simulink model "RealSim_UA_01"  (Simulink 10.0)
settings: Solver=ode1  StartTime=0.0  StopTime=Inf  FixedStep=0.001  RelTol=1e-3  EnableMultiTasking=on
PreLoadFcn:
  | if ~length(which('cmcmd')), cmenv; end
PostLoadFcn:
  | if any(exist('dsrtsu_mdlpostloadfcn', 'file') ~= 0), dsrtsu_mdlpostloadfcn('Execute', bdroot); end
InitFcn:
  | , if any(exist('dsmpb_private', 'file') ~= 0), dsmpb_private('dsmpb_mdlclblib', 'Init', bdroot); end,
undefined symbols (not defined in the file or in its folder): SUMONoDyn_SpeedFromSumo_mps, SUMONoDyn_Time_s
libraries: dsmpblib x7, simulink x4
PreSaveFcn:
  | , if any(exist('dsmpb_private', 'file') ~= 0), dsmpb_private('dsmpb_mdlclblib', 'PreSave', bdroot); end,
CloseFcn:
  | , if any(exist('dsmpb_private', 'file') ~= 0), dsmpb_private('dsmpb_mdlclblib', 'Close', bdroot); end,
settings Model: RTICANMMDATA=struct('GeneralSetupData',struct('modelroot','C:\ORNL\Code\cm10_realsim_UA_proj\src_cm4sl','generalsettings',struct('filesettings',struct('destfolder',struct('Name','RTICANMM_FILES','Check',1),'buildfolder',struct('Name','.','Check',1),'AbsDestfolder',struct('Name','C:\ORNL\Code\cm10_realsim_UA_proj\src_cm4sl\RTICANMM_FILES'),'AbsBuildfolder',struct('Name','C:\ORNL\Code\cm10_realsim_UA_proj\src_cm4sl'))),'options',struct('addpaths',1,'rmpaths',1,'addtrcexclusion',true,'cannavigator',struct('checkmonitoring',0),'show_usrtrc',0,'use_usrtrc',0),'advanced',struct('options',ones(1,100)),'MPSetup',{{}},'RTI',struct('Type','DSRT','Ver','4.2p1','Date','11-Feb-2020'),'modelname','RealSim_UA_01','block','RealSim_UA_01'))  DSRTSU_INTERNAL_RTIFPGA=150  DSMPB_ID_DATA={'3989',struct('BlockId','8a5b4871-e5f6-4132-a2a0-cfdc08ce5a62','SignalIds',{{'f768e98f-af3a-45f5-b8cc-d45140bad16b'}}),'3990',struct('BlockId','8935c71e-55a2-4122-9d8c-9a702d74f083','SignalIds',{{'7beae7fa-5028-4068-8a6f-9b12f3c7f2cd'}}),'3991',struct('BlockId','27d609ef-4027-4865-90b1-f647bdc0d63f','SignalIds',{{'f3b1d4b1-f31f-4d63-9d34-50172078722b','1a0ed1f8-b245-431e-8944-1442373f7090'}}),'3992',struct('BlockId','4d452e4e-1d5d-452d-b859-8d5b2ee4f974','SignalIds',{{'341be20d-510e-43ce-bf93-db3744e3af54','92dd9c2e-376e-43cb-936f-8d32abdccb4f','85825f80-a60d-4715-affe-6d21e145415d','eb0678fd-503c-45b4-9ef8-2c00783b7cf9'}}),'3994',struct('BlockId','13483ad7-c9a4-44e5-950b-a5cc0e7666e2','SignalIds',{{'3f16ee9e-b6cb-44ff-9801-e0155d01597e','6edf7b02-435e-4d6a-b940-049f7bb34941'}}),'3995',struct('BlockId','400b85df-e7bd-4fe3-9c0f-59686a376489','SignalIds',{{'36519bb0-7faf-46a8-b3e5-661b8781a7f8'}}),'4054',struct('BlockId','353e6fb8-1188-4f2a-93b8-42c0e6c342a3','SignalIds',{{'0c3ec644-6183-447e-85a0-984a42e1fc9b'}})}  Creator=fh  LastModifiedBy=Paul_User  ExtModeAutoUpdateStatusClock=off
settings DataIOCC: LimitDataPoints=on  SignalLoggingName=sigsOut
settings OptimizationCC: BlockReduction=off  BooleanDataType=off  ConditionallyExecuteInputs=off  OptimizeBlockIOStorage=off  BufferReuse=off  GlobalBufferReuse=off  ExpressionFolding=off  ExpressionDepthLimit=2147483647  LocalBlockOutputs=off  InitFltsAndDblsToZero=on  LifeSpan=auto  OptimizeDataStoreBuffers=off  BusAssignmentInplaceUpdate=off
settings DebuggingCC: SaveWithParameterizedLinksMsg=none  SignalResolutionControl=TryResolveAllWithWarning  MultiTaskDSMMsg=warning  MultiTaskCondExecSysMsg=none  TasksWithSamePriorityMsg=none  FcnCallInpInsideContextMsg=warning  StateNameClashWarn=warning  SFExecutionAtInitializationDiag=warning
settings HardwareCC: ProdLargestAtomicInteger=Integer  ProdLargestAtomicFloat=Float  ProdIntDivRoundTo=Zero  ProdEndianess=LittleEndian  ProdHWDeviceType=Custom Processor->Custom
settings SFSimCC: MATLABDynamicMemAlloc=off
settings RTWCC: Description=dSPACE Run-Time Target (for VEOS on Windows and ConfigurationDesk)  SystemTargetFile=dsrt.tlc  GenCodeOnly=on  MakeCommand=make_dsrt  TemplateMakefile=dsrt_default_tmf  RTWVerbose=off
settings CodeAppCC: MaxIdLength=63
settings STFCustomTargetCC: ParMdlRefBuildCompliant=on  GRTInterface=off  SystemTargetFile=dsrt.tlc
settings GRTTargetCC: CompOptLevelCompliant=off  ConcurrentExecutionCompliant=off  MatFileLogging=off  CPPClassGenCompliant=off  GRTInterface=off  UseToolchainInfoCompliant=off
settings CustomProperty: DataType=RTWOptions_EnumType__dsrt_1VDFType  Value=TRC
settings EnumStrPairs: String=TRC
settings ConfigComp: CovExternalEMLEnable=off

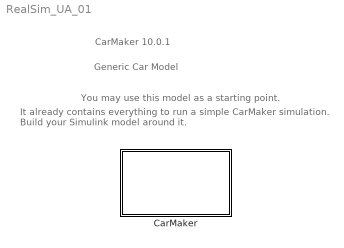
== system RealSim_UA_01 ==
  note: Generic Car Model
  note: You may use this model as a starting point.
  note: It already contains everything to run a simple CarMaker simulation.
      | Build your Simulink model around it.
  note: CarMaker 10.0.1
  CarMaker : Subsystem  TreatAsAtomicUnit=on
      mask Display: image(imread('CarMakerSys.png'));

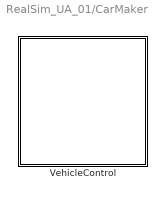
== system RealSim_UA_01/CarMaker ==
  VehicleControl : Subsystem

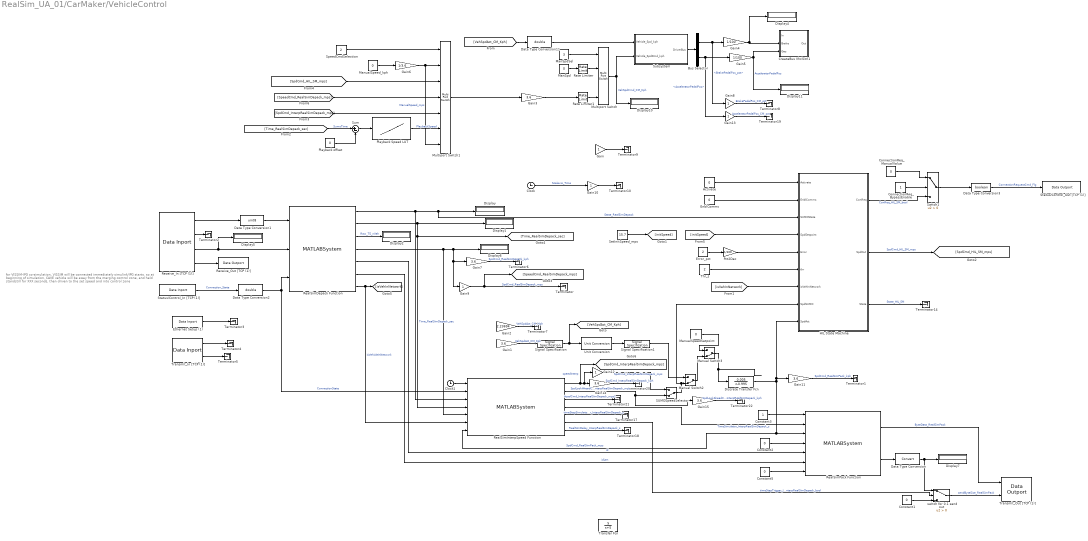
== system RealSim_UA_01/CarMaker/VehicleControl ==
  note: for VISSIM-IPG co-simulation, VISSIM will be connected immediately simulink/IPG starts. so at beginning of simulation, CAVE vehicle will be away from the merging control zone, and held standstill for XXX seconds, then driven to the set speed and into control zone
  Activate : Constant  Value=0
  Bus Selector : BusSelector  OutputSignals=BrakePedalPos_pct,AcceleratorPedalPos
  Clock : Clock
  Clock1 : Clock
  ConnectionReq_BypassEnable : Constant  OutDataTypeStr=boolean
  ConnectionReq_ManualValue : Constant  Value=0  OutDataTypeStr=boolean
  Constant1 : Constant  Value=0
  Constant2 : Constant  Value=0
  Constant3 : Constant
  Constant5 : Constant  Value=0
  CreateBus VhclCtrl1 : Subsystem
  Data Type Conversion : DataTypeConversion
  Data Type Conversion1 : DataTypeConversion  OutDataTypeStr=uint8
  Data Type Conversion11 : DataTypeConversion  OutDataTypeStr=double  LockScale=on
  Data Type Conversion2 : DataTypeConversion  OutDataTypeStr=double
  Data Type Conversion3 : DataTypeConversion  OutDataTypeStr=boolean
  Discrete Transfer Fcn : DiscreteTransferFcn  Numerator=[0.005]  Denominator=[1 -0.995]
  Display{,1..2,4..7,10..11} (9 alike) : Display
  EnblComms : Constant  Value=0
  Error_pct : Constant  Value=2
  Ethernet Setup (1) : dsmpblib/Data Inport  Priority=10000
      settings: SourceProductName=dSPACE Model Interface Blockset
  Gain{,8..10,12..13} (6 alike) : Gain
  Gain{1,3,7,11,14..15} (6 alike) : Gain  Gain=3.6
  Gain2 : Gain  Gain=2.23694
  Gain4 : Gain  Gain=1/100
  Gain5 : Gain  Gain=1/100
  Gain6 : Gain  Gain=1/3.6
  HIL State Machine : Stateflow chart  BlockKeywords=__PRM__SERIALIZED__DATA__:Stateflow Chart,Stateflow Diagram  TreatAsAtomicUnit=on
  ManSpd : Constant  Value=0
  ManSpdSel : Constant  Value=3
  Manual Switch2 : ManualSwitch  CurrentSetting=0
  Manual Switch3 : ManualSwitch  CurrentSetting=0
  ManualSpeedSetpoint : Constant  Value=0
  ManualSpeed_kph : Constant  Value=0
  Multiport Switch : MultiPortSwitch
  Multiport Switch1 : MultiPortSwitch  Inputs=6
  Pct2Dec : Gain  Gain=1/100
  Playback Speed LUT : Lookup_n-D  NumberOfTableDimensions=1  LookupTableObject=''  BreakpointsForDimension1=SUMONoDyn_Time_s  BreakpointsForDimension1FirstPoint=10  BreakpointsForDimension2FirstPoint=10  BreakpointsForDimension1Spacing=12  BreakpointsForDimension2Spacing=12  IndexSearchMethod=Linear search  Table=SUMONoDyn_SpeedFromSumo_mps  InternalRulePriority=Speed  RndMeth=Simplest  InputSameDT=on
  Playback offset : Constant  Value=0
  Rate Limiter : RateLimiter  RisingSlewLimit=10  FallingSlewLimit=-10  SampleTimeMode=inherited
  Rate Limiter1 : RateLimiter  RisingSlewLimit=10  FallingSlewLimit=-20  SampleTimeMode=inherited
  RealSimDepack Function : MATLABSystem  System=RealSimDepack  VehicleMessageFieldDefInputVec=VehicleMessageFieldDefInputVec  SimulateUsing=Code generation
      mask Type: RealSimDepack
      mask Display:
      | disp('RealSimDepack');
      | port_label('input',1,'ByteData');
      | port_label('input',2,'nByte');
      | port_label('input',3,'connectionState');
      | port_label('output',1,'simState');
      | port_label('output',2,'t');
      | port_label('output',3,'nVeh');
      | port_label('output',4,'speed');
      | port_label('output',5,'id');
      | port_label('output',6,'idLen');
      | port_label('output',7,'isVehicleInNetwork');
  RealSimInterpSpeed Function : MATLABSystem  System=RealSimInterpSpeed  initialSpeed=15.7  speedInterpolationMode=0  speedLookAheadHorizon=0.5  speedUpperBound=30  SimulateUsing=Code generation
      mask Type: RealSimInterpSpeed
      mask Display:
      | disp('RealSimInterpSpeed');
      | port_label('input',1,'simulationTime');
      | port_label('input',2,'connectionState');
      | port_label('input',3,'simState');
      | port_label('input',4,'timeReceive');
      | port_label('input',5,'speedReceive');
      | port_label('input',6,'isVehicleInNetwork');
      | port_label('input',7,'speedActual');
      | port_label('output',1,'speedInterp');
      | port_label('output',2,'speedLookAhead');
      | port_label('output',3,'accelerationDesired');
      | port_label('output',4,'timeSimulator');
      | port_label('output',5,'timeStepSimulator');
      | port_label('output',6,'timeStepTrigger');
      | port_label('output',7,'RealSimDelay');
  RealSimPack Function : MATLABSystem  System=RealSimPack  VehicleMessageFieldDefInputVec=VehicleMessageFieldDefInputVec  SimulateUsing=Code generation
      mask Type: RealSimPack
      mask Display:
      | disp('RealSimPack');
      | port_label('input',1,'simState');
      | port_label('input',2,'t');
      | port_label('input',3,'speedDesired');
      | port_label('input',4,'accelerationDesired');
      | port_label('input',5,'id');
      | port_label('input',6,'idLength');
      | port_label('input',7,'activeLaneChange');
      | port_label('output',1,'ByteData');
      | port_label('output',2,'nMsgSize');
  Receive_In [TCP (1)] : dsmpblib/Data Inport  Priority=-10002
      settings: SourceProductName=dSPACE Model Interface Blockset
  Receive_Out [TCP (1)] : dsmpblib/Data Outport  Priority=-10000
      settings: SourceProductName=dSPACE Model Interface Blockset
  SUMOSpeedSelector : ManualSwitch  CurrentSetting=0
  SetInitSpeed_mps : Constant  Value=15.7
  Signal Specification : SignalSpecification  Unit=km/h
  Signal Specification1 : SignalSpecification  Unit=m/s
  SpeedCmdSelection : Constant  Value=2
  Status/Control_In [TCP (1)] : dsmpblib/Data Inport  Priority=-10001
      settings: SourceProductName=dSPACE Model Interface Blockset
  Status/Control_Out [TCP (1)] : dsmpblib/Data Outport  Priority=-10000
      settings: SourceProductName=dSPACE Model Interface Blockset
  Subsystem : Subsystem
  Sum : Sum  Inputs=|+-
  Switch1 : Switch  Criteria=u2 > Threshold
  Terminator{,1..10,14,17..22} (18 alike) : Terminator
  Thr_s : Constant  Value=2
  Transfer Fcn : TransferFcn  Numerator=[5]  Denominator=[1 5]
  Transmit_In [TCP (1)] : dsmpblib/Data Inport  Priority=10000
      settings: SourceProductName=dSPACE Model Interface Blockset
  Transmit_Out [TCP (1)] : dsmpblib/Data Outport  Priority=-10000
      settings: SourceProductName=dSPACE Model Interface Blockset
  Unit Conversion : UnitConversion
  switch for 0.1 send out : Switch  Criteria=u2 > Threshold
  wires:
  Constant5/1 -> RealSimPack Function/7
  Receive_In [TCP (1)]/1 -> Data Type Conversion1/1
  Bus Selector/1 -> Gain8/1, Gain4/1  "<BrakePedalPos_pct>"
  Receive_In [TCP (1)]/4 -> Receive_Out [TCP (1)]/1
  RealSimPack Function/2 -> Data Type Conversion/1
  Constant1/1 -> switch for 0.1 send out/3
  Data Type Conversion/1 -> switch for 0.1 send out/1, Display7/1
  RealSimDepack Function/2 -> Display1/1, [Time_RealSimDepack_sec], RealSimInterpSpeed Function/4  "Time_RealSimDepack_sec"
  Signal Specification1/1 -> Manual Switch2/1
  Transmit_In [TCP (1)]/2 -> Terminator5/1
  [initSpeed] -> HIL State Machine/4(SpdSetpoint)
  EnblComms/1 -> HIL State Machine/2(EnblComms)
  Signal Specification/1 -> [VehSpdAct_CM_Kph], Unit Conversion/1
  Constant3/1 -> RealSimPack Function/1
  Multiport Switch1/1 -> Gain3/1
  Activate/1 -> HIL State Machine/1(Activate)
  Pct2Dec/1 -> HIL State Machine/5(Error)
  Thr_s/1 -> HIL State Machine/6(thr)
  Unit Conversion/1 -> Signal Specification1/1
  Status/Control_In [TCP (1)]/1 -> Data Type Conversion2/1  "Connection_State"
  Gain3/1 -> Rate Limiter1/1
  [VehSpdAct_CM_Kph] -> Data Type Conversion11/1
  SetInitSpeed_mps/1 -> [initSpeed]
  Ethernet Setup (1)/1 -> Terminator3/1
  Transmit_In [TCP (1)]/1 -> Terminator4/1
  Gain5/1 -> CreateBus VhclCtrl1/3(Gas), Display11/1  "AcceleratorPedalPos"
  Error_pct/1 -> Pct2Dec/1
  Gain4/1 -> CreateBus VhclCtrl1/2(Brake), Display4/1
  Multiport Switch/1 -> Display10/1, Subsystem/2(Vehicle_SpdDmd_kph)  "VehSpdCmd_CM_Kph"
  Data Type Conversion11/1 -> Subsystem/1(Vehicle_Spd_kph)
  Subsystem/1(DriverBus) -> Bus Selector/1
  Gain2/1 -> Terminator7/1  "VehSpdAct_CM_Mph"
  Gain9/1 -> [SpeedCmd_RealSimDepack_mps], Terminator/1  "SpdCmd_RealSimDepack_mps"
  Rate Limiter1/1 -> Multiport Switch/4
  Rate Limiter/1 -> Multiport Switch/2
  Gain1/1 -> Signal Specification/1  "VehSpdAct_CM_Kph"
  ManSpd/1 -> Rate Limiter/1
  ManSpdSel/1 -> Multiport Switch/1
  ? -> Multiport Switch/3
  ? -> Gain2/1, Gain1/1  "VehSpdmps"
  Receive_In [TCP (1)]/2 -> Terminator2/1
  Gain7/1 -> Terminator6/1  "SpdCmd_RealSimDepack_kph"
  [SpdCmd_HIL_SM_mps] -> Multiport Switch1/3
  [SpeedCmd_RealSimDepack_mps] -> Multiport Switch1/4
  SpeedCmdSelection/1 -> Multiport Switch1/1
  ? -> Gain/1  "CM_Time"
  ManualSpeed_kph/1 -> Gain6/1
  [Time_RealSimDepack_sec] -> Sum/1  "SumoTime"
  [SpdCmd_InterpRealSimDepack_mps] -> Multiport Switch1/5
  Data Type Conversion3/1 -> Status/Control_Out [TCP (1)]/1  "ConnectionRequestCmd_Flg"
  HIL State Machine/1(ConReq) -> Switch1/3  "ConReq_HIL_SM_bool"
  HIL State Machine/2(SpdOut) -> [SpdCmd_HIL_SM_mps]  "SpdCmd_HIL_SM_mps"
  ConnectionReq_ManualValue/1 -> Switch1/1
  ConnectionReq_BypassEnable/1 -> Switch1/2
  Switch1/1 -> Data Type Conversion3/1
  HIL State Machine/3(State) -> Terminator14/1  "State_HIL_SM"
  Gain/1 -> Terminator9/1
  RealSimDepack Function/1 -> RealSimInterpSpeed Function/3, HIL State Machine/3(SUMOState), Display/1  "State_RealSimDepack"
  RealSimDepack Function/4 -> Display6/1, Gain9/1, Gain7/1, RealSimInterpSpeed Function/5
  RealSimDepack Function/3 -> Display2/1  "Raw_TS_nVeh"
  Gain10/1 -> Terminator10/1
  Clock/1 -> Gain10/1  "Scalexio_Time"
  RealSimPack Function/1 -> Transmit_Out [TCP (1)]/1  "ByteData_RealSimPack"
  switch for 0.1 send out/1 -> Transmit_Out [TCP (1)]/2  "sendByteSize_RealSimPack"
  Data Type Conversion1/1 -> RealSimDepack Function/1
  Receive_In [TCP (1)]/3 -> Display5/1, RealSimDepack Function/2
  RealSimDepack Function/6 -> RealSimPack Function/6  "idLen"
  [isVehInNetwork] -> HIL State Machine/7(isVehInNetwork)
  RealSimDepack Function/5 -> RealSimPack Function/5  "id"
  Constant2/1 -> RealSimPack Function/4
  RealSimDepack Function/7 -> RealSimInterpSpeed Function/6, [isVehInNetwork]  "isVehicleInNetwork"
  Clock1/1 -> RealSimInterpSpeed Function/1
  Manual Switch3/1 -> Discrete Transfer Fcn/1
  RealSimInterpSpeed Function/1 -> [SpdCmd_InterpRealSimDepack_mps], Gain12/1, Gain14/1  "speedInterp"
  Discrete Transfer Fcn/1 -> HIL State Machine/9(SpdAct), Gain11/1, RealSimInterpSpeed Function/7, RealSimPack Function/3  "SpdCmd_RealSimPack_mps"
  RealSimInterpSpeed Function/5 -> Terminator17/1  "timeStepSimulator_InterpRealSimDepack_s"
  RealSimInterpSpeed Function/6 -> switch for 0.1 send out/2  "timeStepTrigger_InterpRealSimDepack_bool"
  RealSimInterpSpeed Function/4 -> RealSimPack Function/2  "TimeSimulator_InterpRealSimDepack_s"
  RealSimInterpSpeed Function/7 -> Terminator18/1  "RealSImDelay_InterpRealSimDepack_s"
  Data Type Conversion2/1 -> RealSimInterpSpeed Function/2, RealSimDepack Function/3  "ConnectionState"
  Gain11/1 -> Terminator1/1  "SpdCmd_RealSimPack_kph"
  Gain12/1 -> SUMOSpeedSelector/1  "SpdCmd_InterpRealSimDepack_mps"
  Gain6/1 -> Multiport Switch1/7, Multiport Switch1/2  "ManualSpeed_mps"
  Gain8/1 -> Terminator8/1  "BrakePedalPos_CM_pct"
  Gain13/1 -> Terminator19/1  "AcceleratorPedalPos_CM_pct"
  Bus Selector/2 -> Gain13/1, Gain5/1  "<AcceleratorPedalPos>"
  Gain14/1 -> Terminator20/1  "SpdCmd_InterpRealSimDepack_kph"
  Playback Speed LUT/1 -> Multiport Switch1/6  "PlaybackSpeed"
  Playback offset/1 -> Sum/2
  Sum/1 -> Playback Speed LUT/1
  Manual Switch2/1 -> Manual Switch3/2
  ManualSpeedSetpoint/1 -> Manual Switch3/1
  RealSimInterpSpeed Function/3 -> Terminator21/1  "AccelCmd_InterpRealSimDepack_mps2"
  SUMOSpeedSelector/1 -> HIL State Machine/8(SpdSUMO), Manual Switch2/2
  RealSimInterpSpeed Function/2 -> Gain15/1, SUMOSpeedSelector/2  "SpdLookAheadCmd_InterpRealSimDepack_mps"
  Gain15/1 -> Terminator22/1  "SpdLookAheadCmd_InterpRealSimDepack_kph"

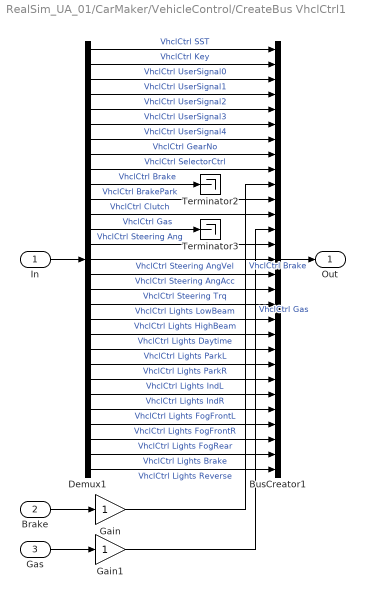
== system RealSim_UA_01/CarMaker/VehicleControl/CreateBus VhclCtrl1 ==
  In : Inport
  Brake : Inport  Port=2
  Gas : Inport  Port=3
  BusCreator1 : BusCreator  Inputs=29
  Demux1 : Demux  Outputs=29
  Gain : Gain
  Gain1 : Gain
  Terminator2 : Terminator
  Terminator3 : Terminator
  Out : Outport
  wires:
  BusCreator1/1 -> Out/1
  In/1 -> Demux1/1
  Brake/1 -> Gain/1
  Gas/1 -> Gain1/1
  Demux1/13 -> Terminator3/1  "VhclCtrl Gas"
  Demux1/10 -> Terminator2/1  "VhclCtrl Brake"
  Demux1/1 -> BusCreator1/1  "VhclCtrl SST"
  Demux1/2 -> BusCreator1/2  "VhclCtrl Key"
  Demux1/3 -> BusCreator1/3  "VhclCtrl UserSignal0"
  Demux1/4 -> BusCreator1/4  "VhclCtrl UserSignal1"
  Demux1/5 -> BusCreator1/5  "VhclCtrl UserSignal2"
  Demux1/6 -> BusCreator1/6  "VhclCtrl UserSignal3"
  Demux1/7 -> BusCreator1/7  "VhclCtrl UserSignal4"
  Demux1/8 -> BusCreator1/8  "VhclCtrl GearNo"
  Demux1/9 -> BusCreator1/9  "VhclCtrl SelectorCtrl"
  Demux1/11 -> BusCreator1/11  "VhclCtrl BrakePark"
  Demux1/12 -> BusCreator1/12  "VhclCtrl Clutch"
  Demux1/14 -> BusCreator1/14  "VhclCtrl Steering Ang"
  Demux1/15 -> BusCreator1/15  "VhclCtrl Steering AngVel"
  Demux1/16 -> BusCreator1/16  "VhclCtrl Steering AngAcc"
  Demux1/17 -> BusCreator1/17  "VhclCtrl Steering Trq"
  Demux1/18 -> BusCreator1/18  "VhclCtrl Lights LowBeam"
  Demux1/19 -> BusCreator1/19  "VhclCtrl Lights HighBeam"
  Demux1/20 -> BusCreator1/20  "VhclCtrl Lights Daytime"
  Demux1/21 -> BusCreator1/21  "VhclCtrl Lights ParkL"
  Demux1/22 -> BusCreator1/22  "VhclCtrl Lights ParkR"
  Demux1/23 -> BusCreator1/23  "VhclCtrl Lights IndL"
  Demux1/24 -> BusCreator1/24  "VhclCtrl Lights IndR"
  Demux1/25 -> BusCreator1/25  "VhclCtrl Lights FogFrontL"
  Demux1/26 -> BusCreator1/26  "VhclCtrl Lights FogFrontR"
  Demux1/27 -> BusCreator1/27  "VhclCtrl Lights FogRear"
  Demux1/28 -> BusCreator1/28  "VhclCtrl Lights Brake"
  Demux1/29 -> BusCreator1/29  "VhclCtrl Lights Reverse"
  Gain/1 -> BusCreator1/10  "VhclCtrl Brake"
  Gain1/1 -> BusCreator1/13  "VhclCtrl Gas"

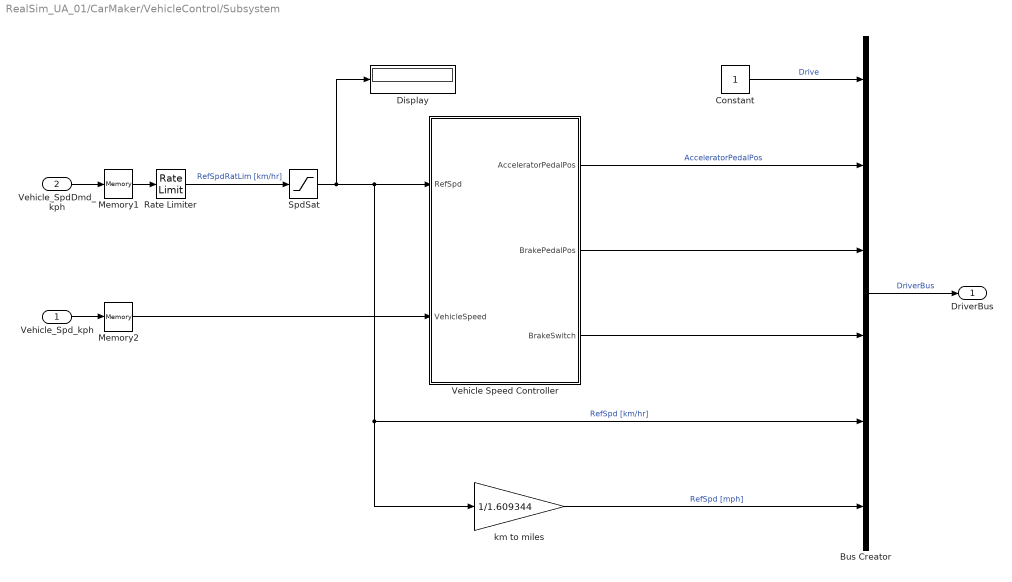
== system RealSim_UA_01/CarMaker/VehicleControl/Subsystem ==
  Vehicle_Spd_kph : Inport
  Vehicle_SpdDmd_kph : Inport  Port=2
  Bus Creator : BusCreator  Inputs=6
  Constant : Constant
  Display : Display
  Memory1 : Memory
  Memory2 : Memory
  Rate Limiter : RateLimiter  RisingSlewLimit=10.8  FallingSlewLimit=-14.4  SampleTimeMode=inherited
  SpdSat : Saturate  UpperLimit=190  LowerLimit=-5
  Vehicle Speed Controller : Subsystem
  km to miles : Gain  Gain=1/1.609344
  DriverBus : Outport
  wires:
  Vehicle_SpdDmd_kph/1 -> Memory1/1
  Constant/1 -> Bus Creator/1  "Drive"
  Vehicle Speed Controller/3(BrakeSwitch) -> Bus Creator/4
  SpdSat/1 -> Display/1, Vehicle Speed Controller/1(RefSpd), km to miles/1, Bus Creator/5  "RefSpd [km/hr]"
  Vehicle Speed Controller/2(BrakePedalPos) -> Bus Creator/3
  Bus Creator/1 -> DriverBus/1  "DriverBus"
  Vehicle_Spd_kph/1 -> Memory2/1
  km to miles/1 -> Bus Creator/6  "RefSpd [mph]"
  Memory1/1 -> Rate Limiter/1
  Memory2/1 -> Vehicle Speed Controller/2(VehicleSpeed)
  Rate Limiter/1 -> SpdSat/1  "RefSpdRatLim [km/hr]"
  Vehicle Speed Controller/1(AcceleratorPedalPos) -> Bus Creator/2  "AcceleratorPedalPos"

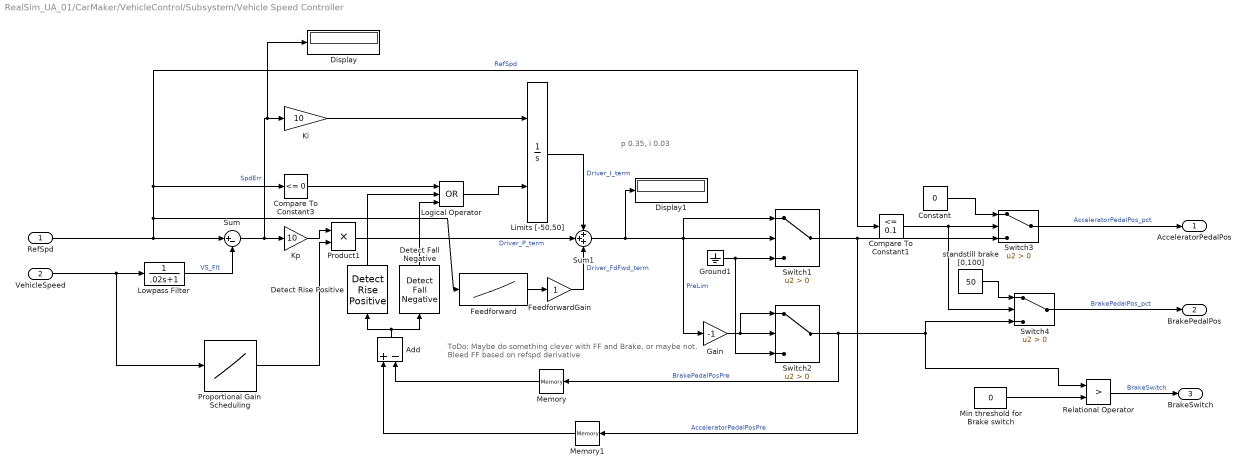
== system RealSim_UA_01/CarMaker/VehicleControl/Subsystem/Vehicle Speed Controller ==
  note: ToDo: Maybe do something clever with FF and Brake, or maybe not.
      | Bleed FF based on refspd derivative
  note: p 0.35, i 0.03
  RefSpd : Inport
  VehicleSpeed : Inport  Port=2
  Add : Sum  Inputs=+-
  Compare To Constant1 : simulink/Logic and Bit Operations/Compare To Constant  relop=<=  const=0.1  OutDataTypeStr=boolean  ZeroCross=off
  Compare To Constant3 : simulink/Logic and Bit Operations/Compare To Constant  relop=<=  const=0  OutDataTypeStr=boolean  ZeroCross=off
  Constant : Constant  Value=0
  Detect Fall Negative : simulink/Logic and Bit Operations/Detect Fall Negative  vinit=0  OutDataTypeStr=boolean
      settings: SourceProductName=Simulink  SourceProductBaseCode=SL
  Detect Rise Positive : simulink/Logic and Bit Operations/Detect Rise Positive  vinit=0  OutDataTypeStr=boolean
  Display : Display
  Display1 : Display
  Feedforward : Lookup_n-D  NumberOfTableDimensions=1  BreakpointsForDimension1="[0 10    20    30    40    50    60    70    80    90   100   110   120   130   140   150   160]"  Table="[0 2.6021    4.7790    6.8575    8.1555    9.4176   10.7914   12.3245   14.1570   15.9699   17.4605   19.0355   21.3079   22.8407   25.3373   26.9453   28.6975]"  ExtrapMethod=Clip  InternalRulePriority=Speed  RndMeth=Simplest  InputSameDT=on
  FeedforwardGain : Gain
  Gain : Gain  Gain=-1
  Ground1 : Ground
  Ki : Gain  Gain=10
  Kp : Gain  Gain=10
  Limits [-50,50] : Integrator  ExternalReset=either  LimitOutput=on  UpperSaturationLimit=50  LowerSaturationLimit=-50
  Logical Operator : Logic  Operator=OR  Inputs=3  AllPortsSameDT=off  OutDataTypeStr=boolean
  Lowpass Filter : TransferFcn  Denominator=[.02 1]
  Memory : Memory
  Memory1 : Memory
  Min threshold for Brake switch : Constant  Value=0
  Product1 : Product  RndMeth=Zero
  Proportional Gain Scheduling : Lookup_n-D  NumberOfTableDimensions=1  BreakpointsForDimension1=[ 0 30 70]  IndexSearchMethod=Linear search  BeginIndexSearchUsingPreviousIndexResult=on  Table=[1 1 1]  ExtrapMethod=Clip  UseLastTableValue=on  RndMeth=Simplest  InputSameDT=on
  Relational Operator : RelationalOperator  Operator=>  OutDataTypeStr=boolean  RndMeth=Nearest
  Sum : Sum  Inputs=|+-
  Sum1 : Sum  Inputs=+++
  Switch{1..4} (4 alike) : Switch  Criteria=u2 > Threshold
  standstill brake [0,100] : Constant  Value=50
  AcceleratorPedalPos : Outport  VectorParamsAs1DForOutWhenUnconnected=off
  BrakePedalPos : Outport  Port=2  VectorParamsAs1DForOutWhenUnconnected=off
  BrakeSwitch : Outport  Port=3  VectorParamsAs1DForOutWhenUnconnected=off
  wires:
  Kp/1 -> Product1/1
  Min threshold for Brake switch/1 -> Relational Operator/2
  Switch1/1 -> Switch3/3, Memory1/1  "AcceleratorPedalPosPre"
  RefSpd/1 -> Feedforward/1, Compare To Constant1/1, Compare To Constant3/1, Sum/1  "RefSpd"
  Sum/1 -> Kp/1, Display/1, Ki/1  "SpdErr"
  Limits [-50,50]/1 -> Sum1/1  "Driver_I_term"
  VehicleSpeed/1 -> Proportional Gain Scheduling/1, Lowpass Filter/1
  Switch2/1 -> Switch4/3, Relational Operator/1, Memory/1  "BrakePedalPosPre"
  Lowpass Filter/1 -> Sum/2  "VS_Flt"
  Relational Operator/1 -> BrakeSwitch/1  "BrakeSwitch"
  Sum1/1 -> Display1/1, Gain/1, Switch1/1, Switch1/2  "PreLim"
  Ki/1 -> Limits [-50,50]/1
  Ground1/1 -> Switch2/3, Switch1/3
  Gain/1 -> Switch2/1, Switch2/2
  Logical Operator/1 -> Limits [-50,50]/2
  Compare To Constant3/1 -> Logical Operator/1
  Detect Rise Positive/1 -> Logical Operator/2
  Detect Fall Negative/1 -> Logical Operator/3
  Add/1 -> Detect Fall Negative/1, Detect Rise Positive/1
  Memory/1 -> Add/2
  Memory1/1 -> Add/1
  Compare To Constant1/1 -> Switch3/2, Switch4/2
  Switch3/1 -> AcceleratorPedalPos/1  "AcceleratorPedalPos_pct"
  Constant/1 -> Switch3/1
  standstill brake [0,100]/1 -> Switch4/1
  Switch4/1 -> BrakePedalPos/1  "BrakePedalPos_pct"
  Proportional Gain Scheduling/1 -> Product1/2
  Product1/1 -> Sum1/2  "Driver_P_term"
  Feedforward/1 -> FeedforwardGain/1
  FeedforwardGain/1 -> Sum1/3  "Driver_FdFwd_term"

== stateflow chart CarMaker/VehicleControl/HIL State Machine ==
  state Start
    en:
    SpdOut = 0;
    ConReq = 0;
    State = 0;
  state Stop
    du:
    ConReq = 0;
    State = 6;
  state Driving
    state BringUpToSpd
      du:
      SpdOut = SpdSetpoint;
      ConReq = 0;
      State = 1;
    state RegularSimulation
      du:
      SpdOut = SpdSUMO;
      ConReq = 1;
      State = 5;
    state WaitForTrafficLayer
      du:
      SpdOut = SpdSetpoint;
      ConReq = 1;
      State = 3;
    state Ready
      du:
      SpdOut = SpdSetpoint;
      ConReq = 0;
      State = 2;
    state WaitForEGOVehInNetwork
      du:
      SpdOut = SpdSetpoint;
      ConReq = 1;
      State = 4;
    (default) -> BringUpToSpd
    WaitForEGOVehInNetwork -> RegularSimulation : [isVehInNetwork>0]
    BringUpToSpd -> (junction 11) : [SpdAct > (SpdSetpoint - SpdSetpoint*Error) && ...
        | SpdAct < (SpdSetpoint + SpdSetpoint*Error)]
        | {State = 1.5}
    WaitForTrafficLayer -> WaitForEGOVehInNetwork : [SUMOState==1]
    Ready -> WaitForTrafficLayer : [EnblComms]
    (junction 11) -> Ready : [after(thr,sec)]
  Stop -> Start : [after(5,sec)]
  (default) -> Start
  Start -> Driving : [Activate]
  RegularSimulation -> Stop : [ ~EnblComms ]
  Driving -> Stop [order 2] : [SUMOState == 255]
  Driving -> Start [order 1] : [~Activate ]
  data: Activate input double; EnblComms input double; SUMOState input double; SpdSetpoint input double; Error input double; thr input double; isVehInNetwork input double; SpdSUMO input double; SpdAct input double; ConReq output boolean; SpdOut output double; State output double
